simulink model "RBT_simulink"  (R2022b)
settings: Solver=VariableStepAuto  StartTime=0.0  StopTime=10.0  RelTol=1e-3
model workspace (MAT data in the model file):
  T = Simulink.Parameter
  T.DataType = 'auto'
  T.Complexity = 'real'
  T.Dimensions = [0 0]
  Ts = 1
libraries: simulink x2
settings Model: NumberOfSteps=10  Creator=Karthik Mothiki  LastModifiedBy=Karthik Mothiki

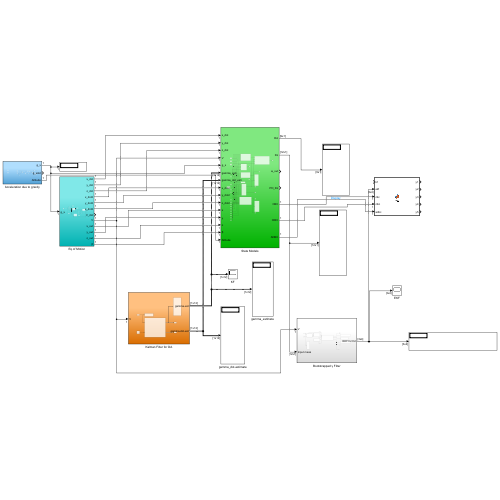
[thumbnail: Simulink's stored preview of the top-level diagram]
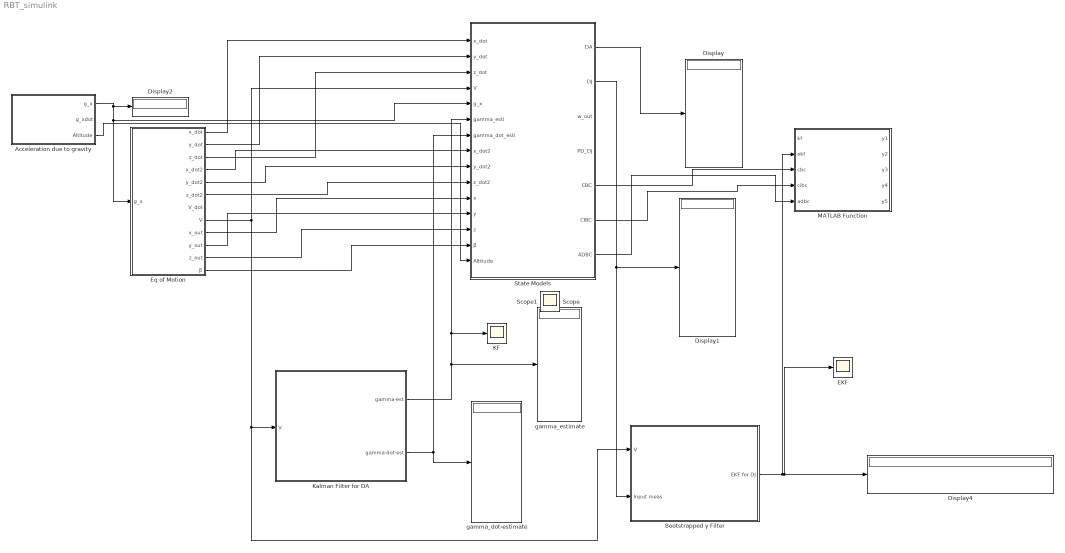
== system RBT_simulink ==
  Acceleration due to gravity : Subsystem
  Bootstrapped γ Filter : Subsystem
  Display{,1..2,4} (4 alike) : Display
  EKF : Scope
  Eq of Motion : Subsystem
  KF : Scope
  Kalman Filter for DA : Subsystem
  MATLAB Function : MATLAB Function  TreatAsAtomicUnit=on
  State Models : Subsystem
  gamma_dot-estimate : Display
  gamma_estimate : Display
  Scope : Scope
  Scope1 : Scope
  wires:
  Eq of Motion/4(x_dot2) -> State Models/8(x_dot2)
  Eq of Motion/5(y_dot2) -> State Models/9(y_dot2)
  Eq of Motion/6(z_dot2) -> State Models/10(z_dot2)
  Acceleration due to gravity/1(g_x) -> State Models/5(g_x), Eq of Motion/1(g_x), Display2/1
  Eq of Motion/1(x_dot) -> State Models/1(x_dot)
  Eq of Motion/2(y_dot) -> State Models/2(y_dot)
  Eq of Motion/3(z_dot) -> State Models/3(z_dot)
  Eq of Motion/11(z_out) -> State Models/13(z)
  Eq of Motion/10(y_out) -> State Models/12(y)
  Eq of Motion/9(x_out) -> State Models/11(x)
  Eq of Motion/8(V) -> Kalman Filter for DA/1(V), Bootstrapped γ Filter/1(V), State Models/4(V)
  Kalman Filter for DA/1(gamma-est) -> State Models/6(gamma_esti), KF/1, gamma_estimate/1
  Kalman Filter for DA/2(gamma-dot-est) -> State Models/7(gamma_dot_esti), gamma_dot-estimate/1
  State Models/1(DA) -> Display/1
  State Models/2(DJ) -> Bootstrapped γ Filter/2(Input meas), Display1/1
  Bootstrapped γ Filter/1(EKF for DJ) -> Display4/1, EKF/1, MATLAB Function/2(ekf)
  Eq of Motion/12(β) -> State Models/14(β)
  Acceleration due to gravity/3(Altitude) -> State Models/15(Altitude)
  State Models/5(CBC) -> MATLAB Function/3(cbc)
  State Models/6(CIBC) -> MATLAB Function/4(cibc)
  State Models/7(ADBC) -> MATLAB Function/5(adbc)

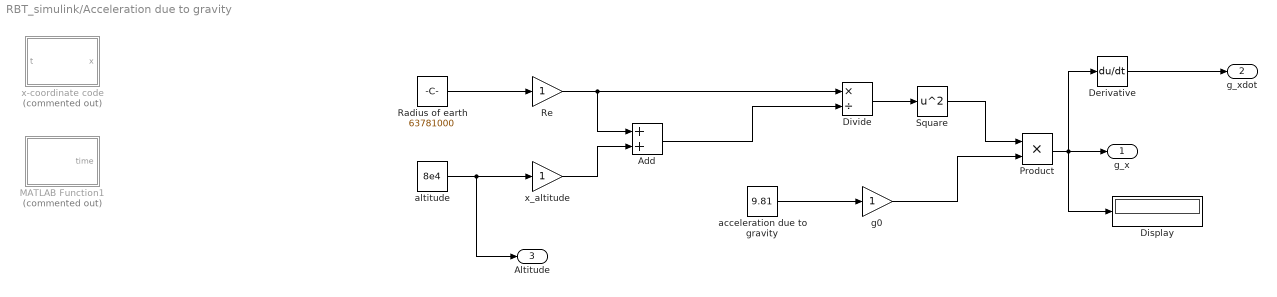
== system RBT_simulink/Acceleration due to gravity ==
  Add : Sum
  Derivative : Derivative
  Display : Display
  Divide : Product  Inputs=*/  RndMeth=Zero  SaturateOnIntegerOverflow=on
  MATLAB Function1 : MATLAB Function  Commented=on  TreatAsAtomicUnit=on
  Product : Product
  Radius of earth : Constant  Value=63781000
  Re : Gain
  Square : Math  Operator=square
  acceleration due to gravity : Constant  Value=9.81
  altitude : Constant  Value=8e4
  g0 : Gain
  x-coordinate code : MATLAB Function  Commented=on  TreatAsAtomicUnit=on
  x_altitude : Gain
  g_x : Outport
  g_xdot : Outport  Port=2
  Altitude : Outport  Port=3
  wires:
  Radius of earth/1 -> Re/1
  altitude/1 -> Altitude/1, x_altitude/1
  x_altitude/1 -> Add/2
  Re/1 -> Divide/1, Add/1
  Add/1 -> Divide/2
  Divide/1 -> Square/1
  acceleration due to gravity/1 -> g0/1
  g0/1 -> Product/2
  Square/1 -> Product/1
  Product/1 -> Display/1, Derivative/1, g_x/1
  Derivative/1 -> g_xdot/1

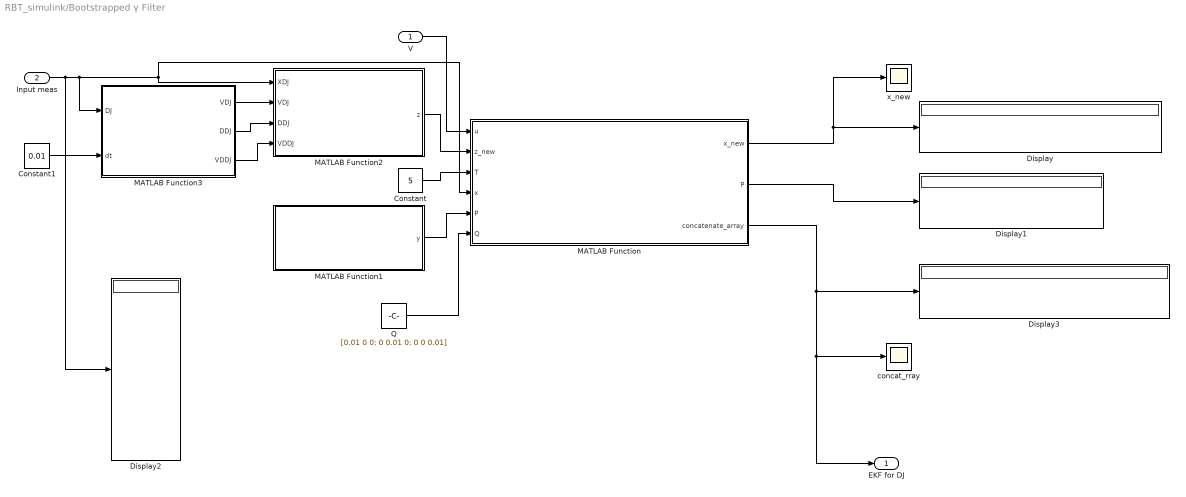
== system RBT_simulink/Bootstrapped γ Filter ==
  V : Inport
  Input meas : Inport  Port=2
  Constant : Constant  Value=5
  Constant1 : Constant  Value=0.01
  Display{,1..3} (4 alike) : Display
  MATLAB Function : MATLAB Function  TreatAsAtomicUnit=on
  MATLAB Function1 : MATLAB Function  TreatAsAtomicUnit=on
  MATLAB Function2 : MATLAB Function  TreatAsAtomicUnit=on
  MATLAB Function3 : MATLAB Function  TreatAsAtomicUnit=on
  Q : Constant  Value=[0.01 0 0; 0 0.01 0; 0 0 0.01]
  concat_rray : Scope
  x_new : Scope
  EKF for DJ : Outport
  wires:
  Input meas/1 -> Display2/1, MATLAB Function2/1(XDJ), MATLAB Function/4(x), MATLAB Function3/1(DJ)
  Constant/1 -> MATLAB Function/3(T)
  V/1 -> MATLAB Function/1(u)
  MATLAB Function3/2(DDJ) -> MATLAB Function2/3(DDJ)
  Constant1/1 -> MATLAB Function3/2(dt)
  MATLAB Function3/3(VDDJ) -> MATLAB Function2/4(VDDJ)
  MATLAB Function1/1(y) -> MATLAB Function/5("P ")
  MATLAB Function3/1(VDJ) -> MATLAB Function2/2(VDJ)
  MATLAB Function2/1(z) -> MATLAB Function/2(z_new)
  MATLAB Function/1(x_new) -> x_new/1, Display/1
  MATLAB Function/2(P) -> Display1/1
  Q/1 -> MATLAB Function/6(Q)
  MATLAB Function/3(concatenate_array) -> Display3/1, EKF for DJ/1, concat_rray/1

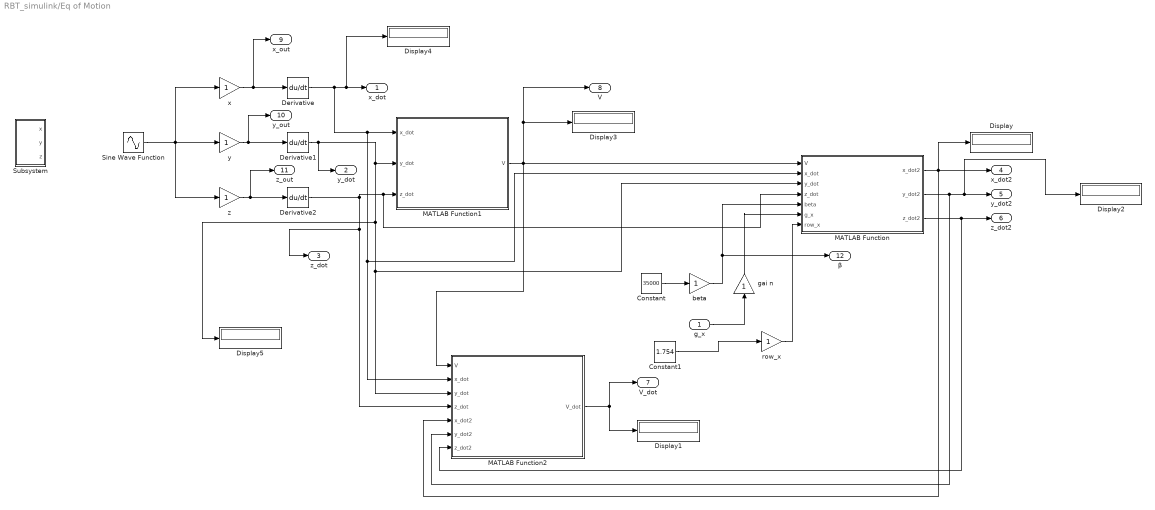
== system RBT_simulink/Eq of Motion ==
  g_x : Inport
  Constant : Constant  Value=35000
  Constant1 : Constant  Value=1.754
  Derivative : Derivative
  Derivative1 : Derivative
  Derivative2 : Derivative
  Display{,1..5} (6 alike) : Display
  MATLAB Function : MATLAB Function  TreatAsAtomicUnit=on
  MATLAB Function1 : MATLAB Function  TreatAsAtomicUnit=on
  MATLAB Function2 : MATLAB Function  TreatAsAtomicUnit=on
  Sine Wave Function : Sin  SampleTime=0
  Subsystem : Subsystem
  beta : Gain
  gai n : Gain
  row_x : Gain
  x : Gain
  y : Gain
  z : Gain
  x_dot : Outport
  y_dot : Outport  Port=2
  z_dot : Outport  Port=3
  x_dot2 : Outport  Port=4
  y_dot2 : Outport  Port=5
  z_dot2 : Outport  Port=6
  V_dot : Outport  Port=7
  V : Outport  Port=8
  x_out : Outport  Port=9
  y_out : Outport  Port=10
  z_out : Outport  Port=11
  β : Outport  Port=12
  wires:
  z/1 -> z_out/1, Derivative2/1
  x/1 -> x_out/1, Derivative/1
  y/1 -> y_out/1, Derivative1/1
  Constant/1 -> beta/1
  g_x/1 -> gai n/1
  Derivative/1 -> Display4/1, x_dot/1, MATLAB Function/2(x_dot), MATLAB Function2/2(x_dot), MATLAB Function1/1(x_dot)
  Derivative1/1 -> y_dot/1, Display5/1, MATLAB Function2/3(y_dot), MATLAB Function/3(y_dot), MATLAB Function1/2(y_dot)
  Derivative2/1 -> MATLAB Function2/4(z_dot), z_dot/1, MATLAB Function/4(z_dot), MATLAB Function1/3(z_dot)
  MATLAB Function1/1(V) -> V/1, Display3/1, MATLAB Function/1(V), MATLAB Function2/1(V)
  beta/1 -> MATLAB Function/5(beta), β/1
  gai n/1 -> MATLAB Function/6(g_x)
  row_x/1 -> MATLAB Function/7(row_x)
  MATLAB Function/1(x_dot2) -> Display/1, MATLAB Function2/5(x_dot2), x_dot2/1
  MATLAB Function/2(y_dot2) -> Display2/1, y_dot2/1, MATLAB Function2/6(y_dot2)
  MATLAB Function/3(z_dot2) -> z_dot2/1, MATLAB Function2/7(z_dot2)
  MATLAB Function2/1(V_dot) -> Display1/1, V_dot/1
  Sine Wave Function/1 -> z/1, x/1, y/1
  Constant1/1 -> row_x/1

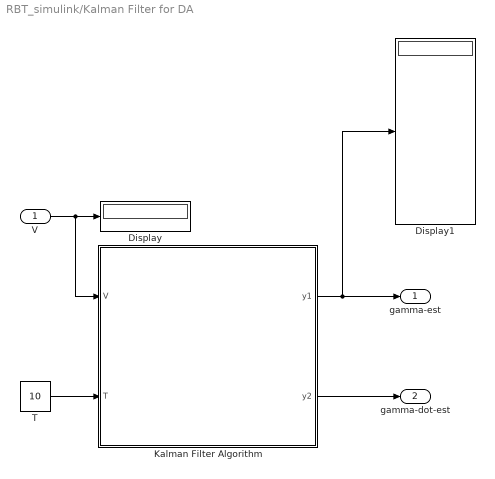
== system RBT_simulink/Kalman Filter for DA ==
  V : Inport
  Display : Display
  Display1 : Display
  Kalman Filter Algorithm : MATLAB Function  TreatAsAtomicUnit=on  SystemSampleTime=0.01
  T : Constant  Value=10
  gamma-est : Outport
  gamma-dot-est : Outport  Port=2
  wires:
  V/1 -> Kalman Filter Algorithm/1(V), Display/1
  T/1 -> Kalman Filter Algorithm/2(T)
  Kalman Filter Algorithm/2(y2) -> gamma-dot-est/1
  Kalman Filter Algorithm/1(y1) -> Display1/1, gamma-est/1

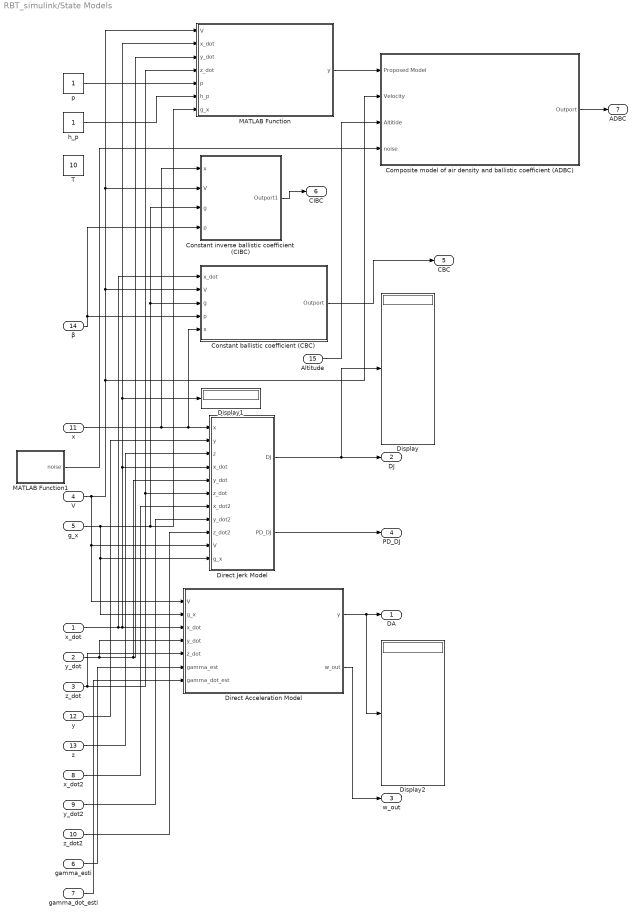
== system RBT_simulink/State Models ==
  x_dot : Inport
  y_dot : Inport  Port=2
  z_dot : Inport  Port=3
  V : Inport  Port=4
  g_x : Inport  Port=5
  gamma_esti : Inport  Port=6
  gamma_dot_esti : Inport  Port=7
  x_dot2 : Inport  Port=8
  y_dot2 : Inport  Port=9
  z_dot2 : Inport  Port=10
  x : Inport  Port=11
  y : Inport  Port=12
  z : Inport  Port=13
  β : Inport  Port=14
  Altitude : Inport  Port=15
  Composite model of air density and ballistic coefficient (ADBC) : Subsystem
  Constant ballistic coefficient (CBC) : Subsystem
  Constant inverse ballistic coefficient (CIBC) : Subsystem
  Direct Acceleration Model : Subsystem
  Direct Jerk Model : Subsystem
  Display : Display
  Display1 : Display
  Display2 : Display
  MATLAB Function : MATLAB Function  TreatAsAtomicUnit=on
  MATLAB Function1 : MATLAB Function  TreatAsAtomicUnit=on
  T : Constant  Value=10
  h_p : Constant
  p : Constant
  DA : Outport
  DJ : Outport  Port=2
  w_out : Outport  Port=3
  PD_DJ : Outport  Port=4
  CBC : Outport  Port=5
  CIBC : Outport  Port=6
  ADBC : Outport  Port=7
  wires:
  p/1 -> MATLAB Function/5(p)
  V/1 -> Direct Jerk Model/10(V), Direct Acceleration Model/1(V), MATLAB Function/1(V), Constant inverse ballistic coefficient (CIBC)/2(V), Constant ballistic coefficient (CBC)/2(V), Composite model of air density and ballistic coefficient (ADBC)/2(Velocity)
  x/1 -> Constant inverse ballistic coefficient (CIBC)/1(x), Constant ballistic coefficient (CBC)/5(x), Direct Jerk Model/1(x)
  y_dot2/1 -> Direct Jerk Model/8(y_dot2)
  g_x/1 -> Direct Acceleration Model/2(g_x), Direct Jerk Model/11(g_x), Constant ballistic coefficient (CBC)/3(g), Constant inverse ballistic coefficient (CIBC)/3(g), MATLAB Function/7(g_x)
  h_p/1 -> MATLAB Function/6(h_p)
  β/1 -> Constant ballistic coefficient (CBC)/4(p), Constant inverse ballistic coefficient (CIBC)/4(p)
  MATLAB Function1/1(noise) -> Composite model of air density and ballistic coefficient (ADBC)/4(noise)
  x_dot/1 -> Constant ballistic coefficient (CBC)/1(x_dot), Display1/1, MATLAB Function/2(x_dot), Direct Jerk Model/4(x_dot), Direct Acceleration Model/3(x_dot)
  y_dot/1 -> MATLAB Function/3(y_dot), Direct Jerk Model/5(y_dot), Direct Acceleration Model/4(y_dot)
  z_dot/1 -> Direct Jerk Model/6(z_dot), MATLAB Function/4(z_dot), Direct Acceleration Model/5(z_dot)
  y/1 -> Direct Jerk Model/2(y)
  MATLAB Function/1(y) -> Composite model of air density and ballistic coefficient (ADBC)/1(Proposed Model)
  x_dot2/1 -> Direct Jerk Model/7(x_dot2)
  z/1 -> Direct Jerk Model/3(z)
  z_dot2/1 -> Direct Jerk Model/9(z_dot2)
  gamma_esti/1 -> Direct Acceleration Model/6(gamma_est)
  gamma_dot_esti/1 -> Direct Acceleration Model/7(gamma_dot_est)
  Direct Jerk Model/2(PD_DJ) -> PD_DJ/1
  Altitude/1 -> Composite model of air density and ballistic coefficient (ADBC)/3(Altitide)
  Direct Jerk Model/1(DJ) -> Display/1, DJ/1
  Direct Acceleration Model/1(y) -> Display2/1, DA/1
  Direct Acceleration Model/2(w_out) -> w_out/1
  Composite model of air density and ballistic coefficient (ADBC)/1(Outport) -> ADBC/1
  Constant inverse ballistic coefficient (CIBC)/1(Outport1) -> CIBC/1
  Constant ballistic coefficient (CBC)/1(Outport) -> CBC/1

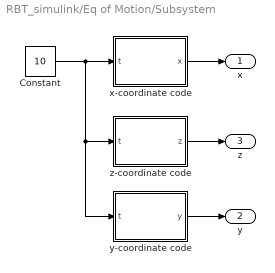
== system RBT_simulink/Eq of Motion/Subsystem ==
  Constant : Constant  Value=10
  x-coordinate code : MATLAB Function  TreatAsAtomicUnit=on
  y-coordinate code : MATLAB Function  TreatAsAtomicUnit=on
  z-coordinate code : MATLAB Function  TreatAsAtomicUnit=on
  x : Outport
  y : Outport  Port=2
  z : Outport  Port=3
  wires:
  Constant/1 -> z-coordinate code/1(t), y-coordinate code/1(t), x-coordinate code/1(t)
  y-coordinate code/1(y) -> y/1
  x-coordinate code/1(x) -> x/1
  z-coordinate code/1(z) -> z/1

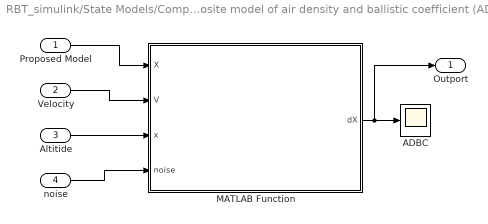
== system RBT_simulink/State Models/Composite model of air density and ballistic coefficient (ADBC) ==
  Proposed Model : Inport
  Velocity : Inport  Port=2
  Altitide : Inport  Port=3
  noise : Inport  Port=4
  ADBC : Scope
  MATLAB Function : MATLAB Function  TreatAsAtomicUnit=on
  Outport : Outport
  wires:
  Proposed Model/1 -> MATLAB Function/1(X)
  Altitide/1 -> MATLAB Function/3(x)
  Velocity/1 -> MATLAB Function/2(V)
  MATLAB Function/1(dX) -> Outport/1, ADBC/1
  noise/1 -> MATLAB Function/4(noise)

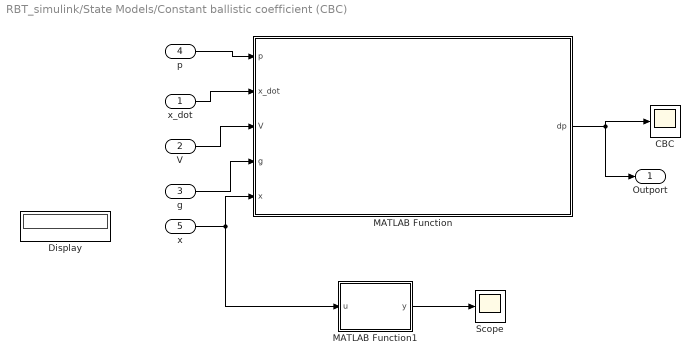
== system RBT_simulink/State Models/Constant ballistic coefficient (CBC) ==
  x_dot : Inport
  V : Inport  Port=2
  g : Inport  Port=3
  p : Inport  Port=4
  x : Inport  Port=5
  CBC : Scope
  Display : Display
  MATLAB Function : MATLAB Function  TreatAsAtomicUnit=on
  MATLAB Function1 : MATLAB Function  TreatAsAtomicUnit=on
  Scope : Scope
  Outport : Outport
  wires:
  x_dot/1 -> MATLAB Function/2(x_dot)
  V/1 -> MATLAB Function/3(V)
  g/1 -> MATLAB Function/4(g)
  p/1 -> MATLAB Function/1(p)
  MATLAB Function/1(dp) -> Outport/1, CBC/1
  x/1 -> MATLAB Function1/1(u), MATLAB Function/5(x)
  MATLAB Function1/1(y) -> Scope/1

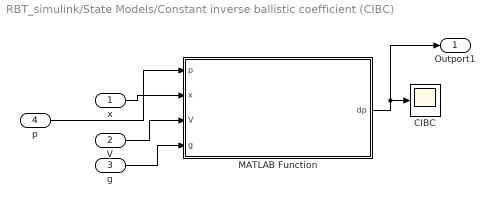
== system RBT_simulink/State Models/Constant inverse ballistic coefficient (CIBC) ==
  x : Inport
  V : Inport  Port=2
  g : Inport  Port=3
  p : Inport  Port=4
  CIBC : Scope
  MATLAB Function : MATLAB Function  TreatAsAtomicUnit=on
  Outport1 : Outport
  wires:
  MATLAB Function/1(dp) -> Outport1/1, CIBC/1
  V/1 -> MATLAB Function/3(V)
  g/1 -> MATLAB Function/4(g)
  x/1 -> MATLAB Function/2(x)
  p/1 -> MATLAB Function/1(p)

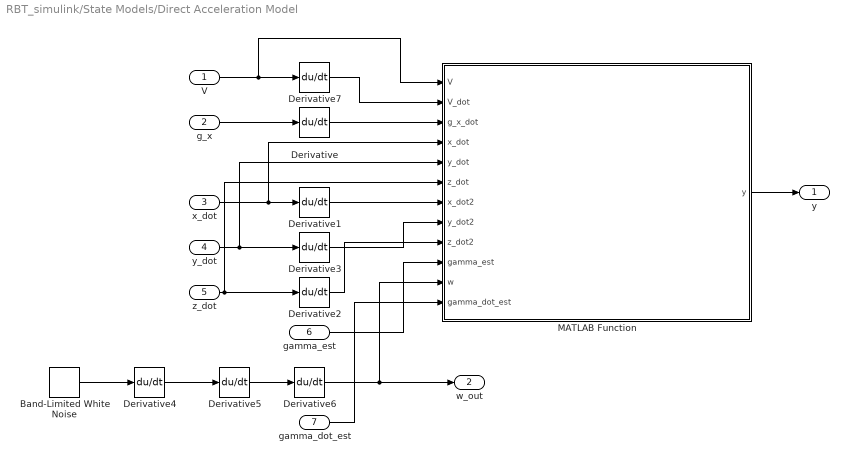
== system RBT_simulink/State Models/Direct Acceleration Model ==
  V : Inport
  g_x : Inport  Port=2
  x_dot : Inport  Port=3
  y_dot : Inport  Port=4
  z_dot : Inport  Port=5
  gamma_est : Inport  Port=6
  gamma_dot_est : Inport  Port=7
  Band-Limited White Noise : simulink/Sources/Band-Limited White Noise  Cov=[0.001]  Ts=0.01  seed=[23341]
  Derivative{,1..7} (8 alike) : Derivative
  MATLAB Function : MATLAB Function  TreatAsAtomicUnit=on
  y : Outport
  w_out : Outport  Port=2
  wires:
  Band-Limited White Noise/1 -> Derivative4/1
  Derivative4/1 -> Derivative5/1
  z_dot/1 -> MATLAB Function/6(z_dot), Derivative2/1
  x_dot/1 -> MATLAB Function/4(x_dot), Derivative1/1
  V/1 -> MATLAB Function/1(V), Derivative7/1
  y_dot/1 -> MATLAB Function/5(y_dot), Derivative3/1
  g_x/1 -> Derivative/1
  Derivative5/1 -> Derivative6/1
  gamma_dot_est/1 -> MATLAB Function/12(gamma_dot_est)
  Derivative7/1 -> MATLAB Function/2(V_dot)
  Derivative/1 -> MATLAB Function/3(g_x_dot)
  Derivative1/1 -> MATLAB Function/7(x_dot2)
  Derivative3/1 -> MATLAB Function/8(y_dot2)
  Derivative2/1 -> MATLAB Function/9(z_dot2)
  gamma_est/1 -> MATLAB Function/10(gamma_est)
  Derivative6/1 -> w_out/1, MATLAB Function/11(w)
  MATLAB Function/1(y) -> y/1

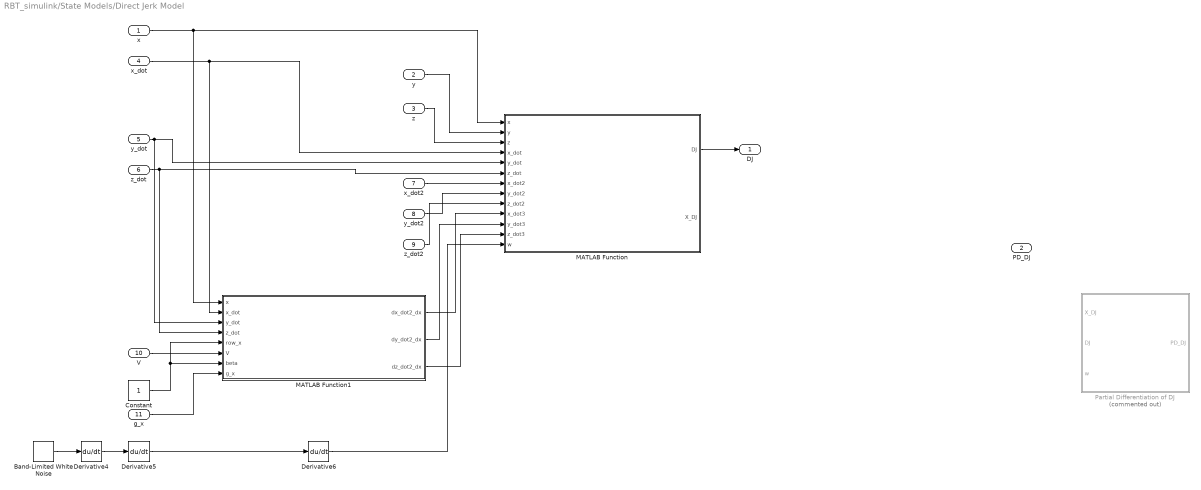
== system RBT_simulink/State Models/Direct Jerk Model ==
  x : Inport
  y : Inport  Port=2
  z : Inport  Port=3
  x_dot : Inport  Port=4
  y_dot : Inport  Port=5
  z_dot : Inport  Port=6
  x_dot2 : Inport  Port=7
  y_dot2 : Inport  Port=8
  z_dot2 : Inport  Port=9
  V : Inport  Port=10
  g_x : Inport  Port=11
  Band-Limited White Noise : simulink/Sources/Band-Limited White Noise  Cov=[0.001]  Ts=0.01  seed=[23341]
  Constant : Constant
  Derivative4 : Derivative
  Derivative5 : Derivative
  Derivative6 : Derivative
  MATLAB Function : MATLAB Function  TreatAsAtomicUnit=on
  MATLAB Function1 : MATLAB Function  TreatAsAtomicUnit=on
  Partial Differentiation of DJ : MATLAB Function  Commented=on  TreatAsAtomicUnit=on
  DJ : Outport
  PD_DJ : Outport  Port=2
  wires:
  Band-Limited White Noise/1 -> Derivative4/1
  Constant/1 -> MATLAB Function1/5(row_x), MATLAB Function1/7(beta)
  V/1 -> MATLAB Function1/6(V)
  Derivative4/1 -> Derivative5/1
  x_dot2/1 -> MATLAB Function/7(x_dot2)
  x/1 -> MATLAB Function/1(x), MATLAB Function1/1(x)
  g_x/1 -> MATLAB Function1/8(g_x)
  x_dot/1 -> MATLAB Function/4(x_dot), MATLAB Function1/2(x_dot)
  y_dot/1 -> MATLAB Function/5(y_dot), MATLAB Function1/3(y_dot)
  z_dot/1 -> MATLAB Function/6(z_dot), MATLAB Function1/4(z_dot)
  Derivative5/1 -> Derivative6/1
  y/1 -> MATLAB Function/2(y)
  z/1 -> MATLAB Function/3(z)
  y_dot2/1 -> MATLAB Function/8(y_dot2)
  z_dot2/1 -> MATLAB Function/9(z_dot2)
  MATLAB Function1/1(dx_dot2_dx) -> MATLAB Function/10(x_dot3)
  MATLAB Function1/2(dy_dot2_dx) -> MATLAB Function/11(y_dot3)
  MATLAB Function1/3(dz_dot2_dx) -> MATLAB Function/12(z_dot3)
  Derivative6/1 -> MATLAB Function/13(w)
  MATLAB Function/1(DJ) -> DJ/1

== matlab function RBT_simulink/Bootstrapped γ Filter/MATLAB Function ==
  data: u input; z_new input; x_new output; T input; P output; x input; P input; Q input; concatenate_array output
function [x_new, P, concatenate_array] = ekf(u, z_new, T, x, P, Q)
%#codegen
% EKF   Extended Kalman Filter for nonlinear dynamic systems
% [x, P] = ekf(f,x,P,h,z,Q,R) returns state estimate, x and state covariance, P
% for nonlinear dynamic system:
% x_k+1 = f(x_k) + w_k
% z_k   = h(x_k) + v_k
% where w ~ N(0,Q) meaning w is gaussian noise with covariance Q
%       v ~ N(0,R) meaning v is gaussian noise with covariance R
%
% Inputs:   u: input vector
%           z: current measurement
%           T: time interval between filter steps
%           x: "a priori" state estimate
%           P: "a priori" estimated state covariance
%
% Output:   x: "a posteriori" state estimate
%           P: "a posteriori" state covariance

% Compute the Jacobian of the state transition function
F = [1 T T^2/2; 0 1 T; 0 0 1];

% Compute the Jacobian of the measurement function
H = [100 0 10];
H_new = [100 0 10; 0 1 0];

% Reshaping the matrices
x_new = reshape(x, 3, 4);
% z_new = reshape(z, 2, 3);

% Compute the measurement noise variance R(k)
r11 = 1;
r22 = 1;
% r11 = (Dx * P(1,1) * Dx') + (Dx * P(1,2) * Dx') + (Dx * P(1,3) * Dx');
% r22 = (Dy * P(2,1) * Dy') + (Dy * P(2,2) * Dy') + (Dy * P(2,3) * Dy');
R = [r11 0; 0 r22];

% Prediction update
x_new = F * x_new;
P = F * P * F' + Q;

% Measurement update
y = z_new - (H * x_new);
S = H_new * P * H_new' + R;
K = P * H_new' / S;
y_new = reshape(y, 2, 48);
some_var = K * y_new;

% Initialize a cell array to store the separate result matrices
num_columns_some_var = size(some_var, 2);
result_matrices = cell(1, num_columns_some_var);

% Perform element-wise addition using a loop
for i = 1:num_columns_some_var
    % Get the i-th column of matrix some_var
    some_var_column = some_var(:, i);

    % Broadcast matrix x_new to match the size of some_var_column
    x_new_broadcasted = repmat(x_new, 1, size(some_var_column, 2));

    % Add the matrices element-wise and store the result
    result_matrices{i} = x_new_broadcasted + some_var_column;
end

x_final = result_matrices;
P = (eye(size(x_final, 1)) - K * H_new) * P;

disp("x_final form EKF of DJ")
disp(x_final)

sz = size(x_final);
disp('size')
disp(sz)

for i = 1:48
    concatenate_array = result_matrices{i};
end

disp("Concat of cell array")
disp(concatenate_array)
end

== matlab function RBT_simulink/Eq of Motion/MATLAB Function2 ==
  data: V input; V_dot output; x_dot input; y_dot input; z_dot input; x_dot2 input; y_dot2 input; z_dot2 input
function V_dot = Velocitydot_fcn(V, x_dot, y_dot, z_dot, x_dot2, y_dot2, z_dot2)

V_dot = ((x_dot * x_dot2) + (y_dot * y_dot2) + (z_dot * z_dot2))/V;

== matlab function RBT_simulink/Eq of Motion/Subsystem/x-coordinate code ==
  data: t input; x output
function x = calculateX(t)
% t: time variable

% Calculate x coordinate as a function of time
x = sin(2*pi*t/10);

disp("X:")
disp(x)
end

== matlab function RBT_simulink/Eq of Motion/Subsystem/y-coordinate code ==
  data: t input; y output
function y = calculateY(t)
% t: time variable

% Calculate y coordinate as a function of time
y = cos(2*pi*t/10);
end

== matlab function RBT_simulink/Eq of Motion/Subsystem/z-coordinate code ==
  data: t input; z output
function z = calculateZ(t)
% t: time variable

% Calculate z coordinate as a function of time
z = t/10;
end

== matlab function RBT_simulink/Eq of Motion/MATLAB Function1 ==
  data: x_dot input; V output; y_dot input; z_dot input
function V = Velocity_fcn(x_dot, y_dot, z_dot)

V = sqrt(x_dot^2 + y_dot^2 + z_dot^2);

== matlab function RBT_simulink/Acceleration due to gravity/MATLAB Function1 ==
  data: time output
function time = timeVector()
% Generate a 1x50 matrix of time values

time = linspace(0, 5, 50); % Adjust the time range as needed
end

== matlab function RBT_simulink/Acceleration due to gravity/x-coordinate code ==
  data: t input; x output
function x = calculateX(t)
% t: time variable

% Calculate x coordinate as a function of time
x = sin(2*pi*t/5);
end

== matlab function RBT_simulink/State Models/Direct Jerk Model/MATLAB Function1 ==
  data: x input; dx_dot2_dx output; x_dot input; y_dot input; z_dot input; row_x input; V input; beta input; g_x input; dy_dot2_dx output; dz_dot2_dx output
function [dx_dot2_dx, dy_dot2_dx, dz_dot2_dx] = calculatePartialDerivatives(x, x_dot, y_dot, z_dot, row_x, V, beta, g_x)
    % Calculate the partial derivatives of x_dot2, y_dot2, and z_dot2 with respect to x
    
    % Calculate intermediate terms
    term1 = ((-0.5 * row_x * x_dot .* V) / beta) - g_x;
    
    % Calculate partial derivatives
    dx_dot2_dx = (-0.5 * row_x * V) / beta;
    dy_dot2_dx = zeros(size(x));
    dz_dot2_dx = zeros(size(x));
    
    % Iterate over each element of x
    for i = 1:numel(x)
        % Calculate partial derivatives for y_dot2 and z_dot2
        dy_dot2_dx(i) = (term1(i) * y_dot(i)) / x_dot(i);
        dz_dot2_dx(i) = (term1(i) * z_dot(i)) / x_dot(i);
    end
end

== matlab function RBT_simulink/State Models/Direct Jerk Model/Partial Differentiation of DJ ==
  data: X_DJ input; PD_DJ output size=[12; 1]; DJ input; w input
function PD_DJ = DirectJerkCalc(X_DJ, DJ, w)

    h = 1e-6; % Step-size for numerical differentiation

    sz = ndims(DJ); % Dimension of DJ model

    for i = 1:sz
        X_DJ(i) = X_DJ(i) + h;
    end

    A = [0 0 0 0 0 0 0 0 0 w w w];
    w_DJ = transpose(A);

    DJ_PD = X_DJ + w_DJ;


    % Computation of Partial Derivatives using finite difference
    for i = 1:sz
        PD_DJ = (DJ_PD(i) - DJ(i)) / h;
    end

%     PD_DJ = X_DJ + w_DJ;

    disp('Partial Differentiation of DJ model, PD_DJ:')
    disp(PD_DJ)

end

== matlab function RBT_simulink/Bootstrapped γ Filter/MATLAB Function1 ==
  data: y output
function y = PosteriorCovariance()
% Initialize the "a priori" state covariance
P = eye(3);

y = P;

== matlab function RBT_simulink/Bootstrapped γ Filter/MATLAB Function2 ==
  data: XDJ input; z output; VDJ input; DDJ input; VDDJ input
function z = generate_measurements(XDJ, VDJ, DDJ, VDDJ)
% GENERATE_MEASUREMENTS Generate measurements for use in Kalman Filter
% z = generate_measurements(XDJ, VDJ, DDJ, VDDJ) returns a 2x1 vector of
% measurements z for use in the Kalman Filter based on the estimated state
% XDJ, its derivative VDJ, its second derivative DDJ, and its third
% derivative VDDJ.
%
% Syntax:
% z = generate_measurements(XDJ, VDJ, DDJ, VDDJ)
%
% Input:
% XDJ - scalar value of estimated state XDJ(k-1|k-1)
% VDJ - scalar value of estimated state derivative VDJ(k-1|k-1)
% DDJ - scalar value of estimated state second derivative DDJ(k-1|k-1)
% VDDJ - scalar value of estimated state third derivative VDDJ(k-1|k-1)
%
% Output:
% z - 2x1 vector of measurements (z_k)

    % Compute measurements based on equation (38)
    z = [XDJ; 0.5 * VDJ .* VDJ + DDJ .* VDJ .* VDJ - 4 * XDJ .* VDDJ + VDJ .* VDJ .* VDJ];
end

== matlab function RBT_simulink/Bootstrapped γ Filter/MATLAB Function3 ==
  data: DJ input; VDJ output; dt input; DDJ output; VDDJ output
function [VDJ, DDJ, VDDJ] = estimate_derivatives(DJ, dt)
% ESTIMATE_DERIVATIVES Estimate derivatives of DJ using finite differences
% [VDJ, DDJ, VDDJ] = estimate_derivatives(DJ, dt) returns the first,
% second, and third derivatives of the given vector DJ using finite
% differences. The time difference between samples is given by dt.
%
% Syntax:
% [VDJ, DDJ, VDDJ] = estimate_derivatives(DJ, dt)
%
% Input:
% DJ - Nx1 vector of DJ values
% dt - scalar value of time difference between samples
%
% Output:
% VDJ - Nx1 vector of estimated first derivatives of DJ
% DDJ - Nx1 vector of estimated second derivatives of DJ
% VDDJ - Nx1 vector of estimated third derivatives of DJ

    % Estimate first derivative using central finite differences
    VDJ = [0; (DJ(3:end) - DJ(1:end-2)) / (2*dt); 0];

    % Estimate second derivative using central finite differences
    DDJ = [0; (DJ(3:end) - 2*DJ(2:end-1) + DJ(1:end-2)) / (dt^2); 0];

    % Estimate third derivative using central finite differences
    VDDJ = [0; 0; (DJ(5:end) - 2*DJ(4:end-1) + 2*DJ(2:end-3) - DJ(1:end-4)) / (2*dt^3); 0; 0];
end

== matlab function RBT_simulink/State Models/Constant ballistic coefficient (CBC)/MATLAB Function ==
  data: p input; x_dot input; V input; g input; dp output; x input
function dp = constant_ballistic_coefficient(p, x_dot, V, g, x)
    % Function to calculate the derivative of p (dp/dt)
    % Inputs:
    % p - Current value of the ballistic coefficient ¯
    % x - Position vector [x, y, z]
    % V - Velocity vector [Vx, Vy, Vz]
    % Output:
    % dp - Derivative of p (dp/dt)

    % Given constants and parameters
    % g = 9.81; % Acceleration due to gravity (m/s^2)
    noise = randn(size(p)); % Additive white Gaussian n
    disp("Noise:")
    disp(noise)

    

    % CBC model: dp/dt = -0.5 * p * Vx - g(x) - 0.5 * noise
    dp = (-0.5 * (p * x_dot) - 0.5*(g * x)) - noise
    % dp = (-0.5 * p * V - g * x_dot) -  noise;
end

== matlab function RBT_simulink/State Models/Constant inverse ballistic coefficient (CIBC)/MATLAB Function ==
  data: dp output; p input; x input; V input; g input
function dp = CIBC_Model(p, x, V, g)
    % Function to calculate the derivative of p (dp/dt)
    % Inputs:
    % t - Time (not used in the CBC model)
    % p - Current value of the ballistic coefficient ¯
    % x - Position vector [x, y, z]
    % V - Velocity vector [Vx, Vy, Vz]
    % Output:
    % dp - Derivative of p (dp/dt)

    % Given constants and parameters
    % g = 9.81; % Acceleration due to gravity (m/s^2)
    noise = randn(size(p)); % Additive white Gaussian n

    % CIBC model: dp/dt = -0.5 * p * Vx - g(x) - 0.5 * noise
    dp = -0.5 * (1/p) * V(1) - g * x(1) - 0.5 * noise;
end

== matlab function RBT_simulink/State Models/Composite model of air density and ballistic coefficient (ADBC)/MATLAB Function ==
  data: dX output; X input; V input; x input; noise input
function dX = ADBC_Model(X, V, x, noise)
    % ADBC model state equations
    % Inputs:
    % t - Time (not used in the ADBC model)
    % X - State vector [x, y, z, x_dot, y_dot, z_dot, gamma]
    % V - Velocity vector [Vx, Vy, Vz]
    % x - Altitude of the target
    % Output:
    % dX - Derivatives of the state variables

    % Given constants and parameters
    g = 9.81; % Acceleration due to gravity (m/s^2)
    h0 = 1.2; % Empirical relation constant for air density at sea level
    k = 0.01; % Empirical relation constant for air density variation
    p0 = 0.5; % Initial value for ¯ at x=0
    p1 = 0.1; % Linear variation coefficient of ¯ with altitude

    % Unpack state variables
    x_pos = X(1);
    y_pos = X(2);
    z_pos = X(3);
    x_dot = X(4);
    y_dot = X(5);
    z_dot = X(6);
    gamma = X(7);

    % Calculate the air density using the empirical relation (7)
    rho = h0 * exp(-k * x);

    % Calculate the dynamics of the new parameter gamma (Equation 9)
    C = k + p1 / (p0 + p1 * x);
    d_gamma = -C * x_dot + noise;

    % Calculate the derivatives of the state variables
    dx_pos = x_dot;
    dy_pos = y_dot;
    dz_pos = z_dot;
    dx_dot = -0.5 * gamma * V - g * x_pos;
    dy_dot = -0.5 * gamma * V;
    dz_dot = -0.5 * gamma * V;

    % Pack the derivatives into the output vector
    % dX = [dx_pos; dy_pos; dz_pos; dx_dot; dy_dot; dz_dot; d_gamma];
    dX = d_gamma
end

== matlab function RBT_simulink/State Models/MATLAB Function1 ==
  data: noise output
function noise = noise_gen()

% Set the parameters for the noise
mean_value = 1e-8;   % Mean of the Gaussian noise
std_deviation =  1e-3;   % Standard deviation of the Gaussian noise
num_samples = 1;  % Number of samples to generate

% Generate white Gaussian noise
noise = mean_value + std_deviation * randn(num_samples, 1);

end

== matlab function RBT_simulink/State Models/Constant ballistic coefficient (CBC)/MATLAB Function1 ==
  data: y output; u input
function y = ConstantBallisticCoefficientModel(u)
    % Parameters
    num_samples = 1000;      % Number of samples
    time_interval = 0.01;   % Time interval between samples
    
    % Generate time values
    t = (0:num_samples-1) * time_interval;
    
    % Constants
    g = 9.81;   % Acceleration due to gravity
    
    % Generate noisy position signal
    noise_level = 0.2;  % Adjust the noise level as needed
    noise = noise_level * randn(1, num_samples);  % Generate random noise
    x = zeros(1, num_samples);
    
    % Initial conditions
    x(1) = 0;   % Initial position
    v = 0;      % Initial velocity
    
    % Simulation loop
    for i = 2:num_samples
        % Calculate acceleration
        a = -0.5 * x(i-1) * v - g;
        
        % Update velocity and position
        v = v + a * time_interval;
        x(i) = x(i-1) + v * time_interval;
        
        % Add noise to position
        x(i) = x(i) + noise(i);
    end
    
    % Output the noisy position signal
    y = x';
end

== matlab function RBT_simulink/MATLAB Function ==
  data: kf input; y1 output; ekf input; cbc input; cibc input; adbc input; y2 output; y3 output; y4 output; y5 output
function [y1, y2, y3, y4, y5] = fcn(kf, ekf, cbc, cibc, adbc)


t = linspace(0, 10, 1000);

y1 = kf(5);
y2 = ekf(5);
y3 = cbc;
y4 = cibc;
y5 = adbc;

grid on

title('Kinematic State Estimation of and RBT using KF & EKF methods')


plot(t, y1)
hold on

plot(t, y2)
hold on

title('Dynamic Properties of CBC, CIBC & ADBC models')

plot(t, y3)
hold on

plot(t, y4)
hold on

plot(t, y5)
hold off

== matlab function RBT_simulink/State Models/MATLAB Function ==
  data: V input; y output; x_dot input; y_dot input; z_dot input; p input; h_p input; g_x input
function y = proposed_model(V, x_dot,y_dot, z_dot, p, h_p, g_x)
%#codegen

w_x_dot2 = 1;
w_y_dot2 = 1;
w_z_dot2 = 1;

A = [x_dot; y_dot; z_dot; (-0.5 * p * x_dot .* V) - g_x; -0.5 * p * y_dot .* V; -0.5 * p * z_dot .* V; h_p];
% A = [1; 1; 1; 1; 1; 1; 1];
B = [0; 0; 0; w_x_dot2; w_y_dot2; w_z_dot2; 0];
y = A + B;

disp('Proposed Model: ')
disp(y)

== matlab function RBT_simulink/Eq of Motion/MATLAB Function ==
  data: V input; x_dot input; y_dot input; z_dot input; x_dot2 output; beta input; g_x input; row_x input; y_dot2 output; z_dot2 output
function [x_dot2, y_dot2, z_dot2] = Eq_of_Motion(V, x_dot, y_dot, z_dot, beta, g_x, row_x)

x_dot2 = ((-0.5 * row_x * x_dot .* V)/beta) - g_x;
y_dot2 = (-0.5 * row_x * y_dot .* V)/beta;
z_dot2 = (-0.5 * row_x * z_dot .* V)/beta;

disp("Velocity, V = ")
disp(V)

disp("x_dot2= ")
disp(x_dot2)
disp("y_dot2= ")
disp(y_dot2)
disp("z_dot2= ")
disp(z_dot2)

% y = [x_dot2; y_dot2; z_dot2];
% disp(y)

== matlab function RBT_simulink/State Models/Direct Acceleration Model/MATLAB Function ==
  settings: updateMethod=DISCRETE  sampleTime=0.1
  data: y output; V input; V_dot input; g_x_dot input; x_dot input; y_dot input; z_dot input; x_dot2 input; y_dot2 input; z_dot2 input; gamma_est input; w input; gamma_dot_est input
function y = Direct_Acceleration(V, V_dot, g_x_dot, x_dot, y_dot, z_dot, x_dot2, y_dot2, z_dot2, gamma_est, w, gamma_dot_est)

% V_dot = diff(V);

% x_dot = ones(1, 50);
% y_dot = ones(1, 50);
% z_dot = ones(1, 50);

w_x_bar = w;
w_y_bar = w;
w_z_bar = w;

T = 10;
for t = 1:T
    f_x_bar = (-0.5 .* gamma_dot_est(t) .* x_dot .* V) + (-0.5 .* gamma_est(t) .* x_dot2 .* V) - 0.5 .* (gamma_est(t) .* x_dot .* V_dot) - g_x_dot;
    f_y_bar = (-0.5 .* gamma_dot_est(t) .* y_dot .* V) + (-0.5 .* gamma_est(t) .* y_dot2 .* V) - 0.5 .* (gamma_est(t) .* y_dot .* V_dot);
    f_z_bar = (-0.5 .* gamma_dot_est(t) .* z_dot .* V) + (-0.5 .* gamma_est(t) .* z_dot2 .* V) - 0.5 .* (gamma_est(t) .* z_dot .* V_dot);
    
    % f_x_bar = 1;
    % f_y_bar = 1;
    % f_z_bar = 1;
    
    fDA_XDA = [x_dot; y_dot; z_dot; x_dot2; y_dot2; z_dot2; f_x_bar; f_y_bar; f_z_bar];
    W_DA = [0; 0; 0; 0; 0; 0; w_x_bar; w_y_bar; w_z_bar];
    
    y = fDA_XDA + W_DA;
    
    disp('Direct Acceleration Model at t = ')
    disp(t)
    disp(y)
end

== matlab function RBT_simulink/State Models/Direct Jerk Model/MATLAB Function ==
  data: x input; y input; z input; DJ output; x_dot input; y_dot input; z_dot input; x_dot2 input; y_dot2 input; z_dot2 input; x_dot3 input; y_dot3 input; z_dot3 input; w input; X_DJ output
function [DJ, X_DJ] = DirectJerk(x, y, z, x_dot, y_dot, z_dot, x_dot2, y_dot2, z_dot2, x_dot3, y_dot3, z_dot3, w)

X_DJ_normal = [x y z x_dot y_dot z_dot x_dot2 y_dot2 z_dot2 x_dot3 y_dot3 z_dot3];
X_DJ = transpose(X_DJ_normal);
A = [0 0 0 0 0 0 0 0 0 w w w];
wDJ = transpose(A);

DJ = X_DJ + wDJ;
disp("DJ Model")
disp(DJ)

== matlab function RBT_simulink/Kalman Filter for DA/Kalman Filter Algorithm ==
  settings: sampleTime=0.01
  data: y1 output size=[1 12]; V input; T input; y2 output size=[1 12]
function [y1, y2] = kalmanFilter(V, T)
    % V: Velocity
    % T: Number of time steps

    disp('Velocity:')    
    disp(V)
    % Generate synthetic data for D (drag) and D_ (drag derivative)
    D_true = zeros(1, 50);
    D_true(1:T/2) = 10;
    D_true((T/2) + 1:end) = 5;
    D_noise = 0.5 * randn(1, 50);
    D = D_true + D_noise;

    D_ = diff(D) ./ diff(1:50); % Compute D_ using finite differences
    D_ = padarray(D_, [0 1], 'replicate', 'post'); % Pad one element at the end
    
    % Bootstrap estimation using Kalman filter
    gamma_est = zeros(1, T);
    gamma_dot_est = zeros(1, T);
    
    % Initial guess for gamma and gamma_dot
    gamma_est(1) = 0.5;
    gamma_dot_est(1) = 0.1;
    
    % Process noise covariance
    Q = diag([0.01, 0.01]);
    
    % Measurement noise covariance
    R = 0.1;

    % Kalman filter loop
    for t = 2:T
        % Prediction step
        gamma_pred = gamma_est(t-1);
        gamma_dot_pred = gamma_dot_est(t-1);
    
        % Compute pseudo measurements
        D_pred = 0.5 * V^2 * gamma_pred;
        D_dot_pred = ((2 * D_pred * gamma_dot_pred) / V^2) - ((4 * D_pred * gamma_dot_pred^2) / V^3);
    
        % Update step
        K = [gamma_dot_pred * V^2 / (2 * D_pred), 0];
        gamma_est(t) = gamma_est(t-1) + K(1) * (D(t) - D_pred);
%         gamma_est(t) = gamma_est(t-1) + K(1) * (D_(t) - D_pred(t));
    
        % Fix indexing for D_
        D_dot_index = min(t, T-1);
        gamma_dot_est(t) = (gamma_dot_pred + K(2) * (D_(D_dot_index) - D_dot_pred));
    end    

    y1 = gamma_est; 
    y2 = gamma_dot_est;

% Plot the estimated values
% figure;
% subplot(2,1,1);
% plot(gamma_est);
% xlabel('Time step');
% ylabel('Estimated gamma');
% 
% subplot(2,1,2);
% plot(gamma_dot_est);
% xlabel('Time step');
% ylabel('Estimated gamma_dot');
